simulink model "lorenz2"  (Simulink 6.0)
settings: Solver=ode23  SolverMode=SingleTasking  StartTime=0.0  StopTime=inf  RelTol=1e-3  AbsTol=1e-6
settings Model: Creator=The MathWorks Inc.  LastModifiedBy=batserve  ExtModeTrigMode=oneshot  ExtModeArmWhenConnect=off  ExtModeAutoUpdateStatusClock=off
settings DataIOCC: ExternalInput=[]  InitialState=[]  LimitDataPoints=off  SaveOutput=off  SaveTime=off
settings OptimizationCC: BooleanDataType=off
settings DebuggingCC: CheckExecutionContextPreStartOutputMsg=on  CheckExecutionContextRuntimeOutputMsg=on  SolverPrmCheckMsg=none  IntegerOverflowMsg=none
settings HardwareCC: TargetUnknown=on

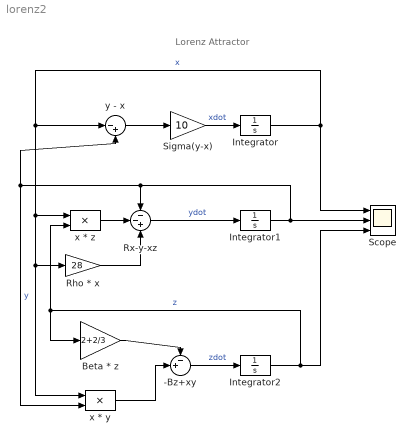
== system lorenz2 ==
  note: Lorenz Attractor
  -Bz+xy : Sum  Inputs=-+|  InputSameDT=on
  Beta * z : Gain  Gain=2+2/3  SaturateOnIntegerOverflow=on
  Integrator : Integrator  InitialCondition=1
  Integrator1 : Integrator  InitialCondition=1
  Integrator2 : Integrator  InitialCondition=1
  Rho * x : Gain  Gain=28  SaturateOnIntegerOverflow=on
  Rx-y-xz : Sum  Inputs=--+  SaturateOnIntegerOverflow=on  InputSameDT=on
  Scope : Scope  NumInputPorts=3
      settings: TickLabels=on  TimeRange=20  YMin=-25~-25~-50  YMax=25~25~50  DataFormat=Array
  Sigma(y-x) : Gain  Gain=10  SaturateOnIntegerOverflow=on
  x * y : Product  SaturateOnIntegerOverflow=on  RndMeth=Zero  InputSameDT=on
  x * z : Product  SaturateOnIntegerOverflow=on  RndMeth=Zero  InputSameDT=on
  y - x : Sum  Inputs=|-+  SaturateOnIntegerOverflow=on  InputSameDT=on
  wires:
  Integrator/1 -> Scope/1, x * y/1, Rho * x/1, x * z/1, y - x/1  "x"
  Integrator1/1 -> Scope/2, y - x/2, x * y/2, Rx-y-xz/1  "y"
  Sigma(y-x)/1 -> Integrator/1  "xdot"
  y - x/1 -> Sigma(y-x)/1
  -Bz+xy/1 -> Integrator2/1  "zdot"
  Beta * z/1 -> -Bz+xy/1
  x * y/1 -> -Bz+xy/2
  Rx-y-xz/1 -> Integrator1/1  "ydot"
  Integrator2/1 -> x * z/2, Beta * z/1, Scope/3  "z"
  x * z/1 -> Rx-y-xz/2
  Rho * x/1 -> Rx-y-xz/3
